simulink model "P_car"  (R2013b)
settings: Solver=ode45  StartTime=0.0  StopTime=10.0  RelTol=1e-3
values from neighbouring files (symbols this model uses):
  g = 9.81    [parameters.m]
  l_p = sqrt(0.115^2 + h_CG^2)    [parameters.m]
  l_w = 0.30    (= 0.3)    [parameters.m]    (also in testing.m = 0.4)
  m_car = 0.7    [dynamics_constants.m]    (also in parameters.m = 1.2)
  pf_mapping_1st_FR = polyfit(alphaF,beta_F,1)    [parameters.m]
  pf_mapping_1st_RR = mean(beta_R)    [parameters.m]
  v_R = 1 + 0.2*randn    [analyze_parameter_impcact.m]    (also in parameters.m = 1)
  w_w = 20    [parameters.m]
  w_z = 0.5    [parameters.m]
settings Model: Creator=daniel  LastModifiedBy=daniel

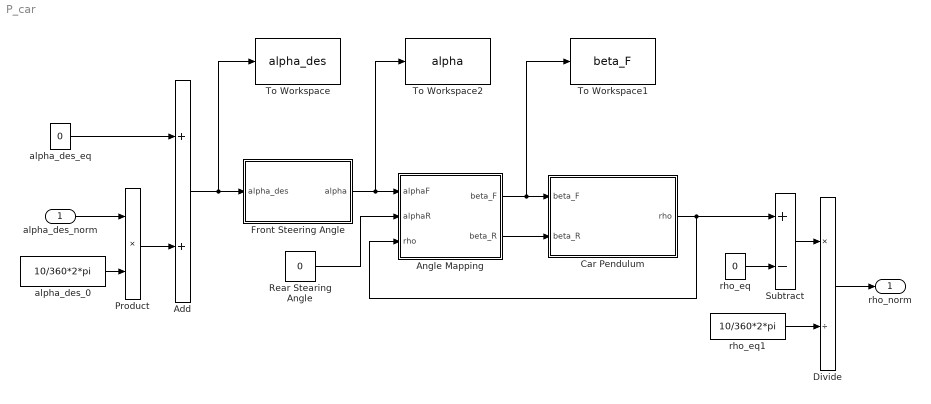
== system P_car ==
  alpha_des_norm : Inport
  Add : Sum
  Angle Mapping : Subsystem
  Car Pendulum : Subsystem
  Divide : Product  Inputs=*/
  Front Steering Angle : Subsystem
  Product : Product
  Rear Stearing Angle : Constant  Value=0
  Subtract : Sum  Inputs=+-
  To Workspace : ToWorkspace  VariableName=alpha_des  SampleTime=-1  SaveFormat=Timeseries
  To Workspace1 : ToWorkspace  VariableName=beta_F  SampleTime=-1  SaveFormat=Timeseries
  To Workspace2 : ToWorkspace  VariableName=alpha  SampleTime=-1  SaveFormat=Timeseries
  alpha_des_0 : Constant  Value=10/360*2*pi
  alpha_des_eq : Constant  Value=0
  rho_eq : Constant  Value=0
  rho_eq1 : Constant  Value=10/360*2*pi
  rho_norm : Outport
  wires:
  Car Pendulum/1(rho) -> Subtract/1, Angle Mapping/3(rho)
  Angle Mapping/2(beta_R) -> Car Pendulum/2(beta_R)
  Rear Stearing Angle/1 -> Angle Mapping/2(alphaR)
  Angle Mapping/1(beta_F) -> To Workspace1/1, Car Pendulum/1(beta_F)
  alpha_des_0/1 -> Product/2
  alpha_des_norm/1 -> Product/1
  Product/1 -> Add/2
  Add/1 -> To Workspace/1, Front Steering Angle/1(alpha_des)
  alpha_des_eq/1 -> Add/1
  rho_eq/1 -> Subtract/2
  Subtract/1 -> Divide/1
  rho_eq1/1 -> Divide/2
  Divide/1 -> rho_norm/1
  Front Steering Angle/1(alpha) -> To Workspace2/1, Angle Mapping/1(alphaF)

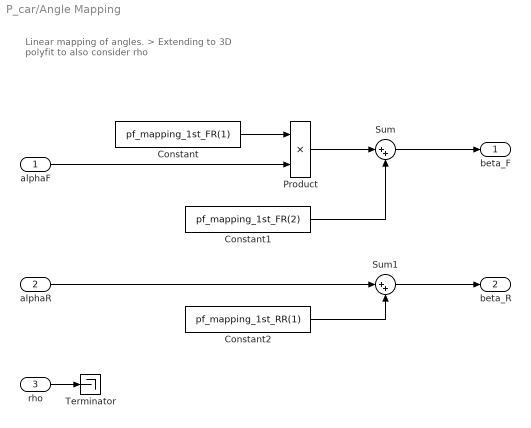
== system P_car/Angle Mapping ==
  note: Linear mapping of angles.
      |
      | > Extending to 3D polyfit to also consider rho
  alphaF : Inport
  alphaR : Inport  Port=2
  rho : Inport  Port=3
  Constant : Constant  Value=pf_mapping_1st_FR(1)
  Constant1 : Constant  Value=pf_mapping_1st_FR(2)
  Constant2 : Constant  Value=pf_mapping_1st_RR(1)
  Product : Product
  Sum : Sum  Inputs=|++
  Sum1 : Sum  Inputs=|++
  Terminator : Terminator
  beta_F : Outport
  beta_R : Outport  Port=2
  wires:
  Constant1/1 -> Sum/2
  Product/1 -> Sum/1
  Constant/1 -> Product/1
  alphaF/1 -> Product/2
  Sum/1 -> beta_F/1
  Sum1/1 -> beta_R/1
  alphaR/1 -> Sum1/1
  Constant2/1 -> Sum1/2
  rho/1 -> Terminator/1

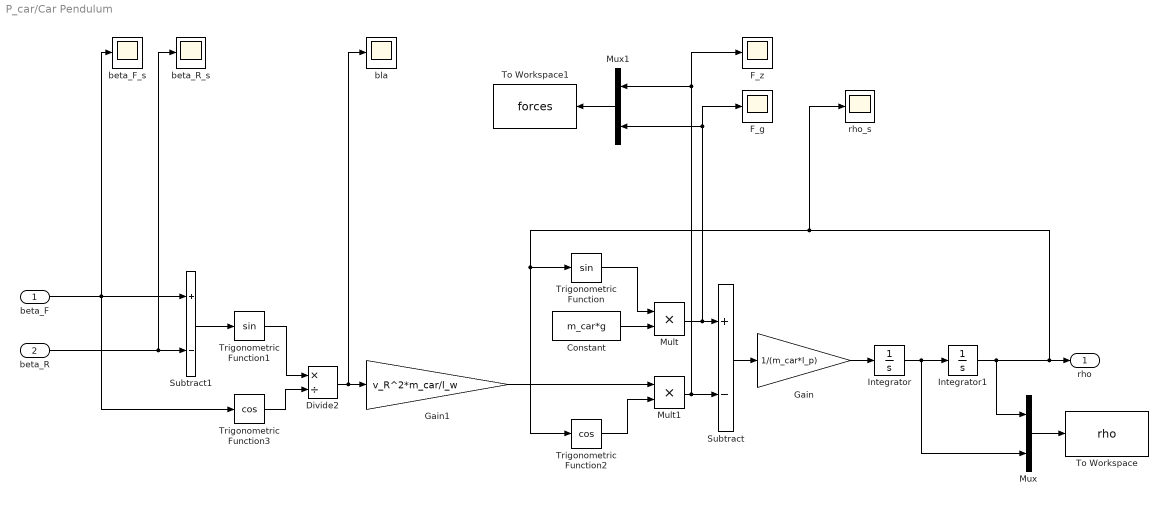
== system P_car/Car Pendulum ==
  beta_F : Inport
  beta_R : Inport  Port=2
  Constant : Constant  Value=m_car*g
  Divide2 : Product  Inputs=*/
  F_g : Scope
      settings: SaveName=ScopeData2
  F_z : Scope
  Gain : Gain  Gain=1/(m_car*l_p)
  Gain1 : Gain  Gain=v_R^2*m_car/l_w
  Integrator : Integrator  ContinuousStateAttributes='rho_dot'
  Integrator1 : Integrator  InitialCondition=2/360*2*pi*0  ContinuousStateAttributes='rho'
  Mult : Product  Inputs=**
  Mult1 : Product  Inputs=**
  Mux : Mux  Inputs=2
  Mux1 : Mux  Inputs=2
  Subtract : Sum  Inputs=+-
  Subtract1 : Sum  Inputs=+-
  To Workspace : ToWorkspace  VariableName=rho  SampleTime=-1  SaveFormat=Timeseries
  To Workspace1 : ToWorkspace  VariableName=forces  SampleTime=-1  SaveFormat=Timeseries
  Trigonometric Function : Trigonometry
  Trigonometric Function1 : Trigonometry
  Trigonometric Function2 : Trigonometry  Operator=cos
  Trigonometric Function3 : Trigonometry  Operator=cos
  beta_F_s : Scope
      settings: SaveName=ScopeData7
  "beta_R_s " : Scope
      settings: SaveName=ScopeData9
  bla : Scope
      settings: SaveName=ScopeData10
  rho_s : Scope
      settings: SaveName=ScopeData3
  rho : Outport
  wires:
  Integrator/1 -> Mux/2, Integrator1/1
  Mult1/1 -> F_z/1, Mux1/1, Subtract/2
  Mult/1 -> F_g/1, Mux1/2, Subtract/1
  beta_F/1 -> Trigonometric Function3/1, beta_F_s/1, Subtract1/1
  beta_R/1 -> "beta_R_s "/1, Subtract1/2
  Trigonometric Function1/1 -> Divide2/1
  Divide2/1 -> bla/1, Gain1/1
  Gain/1 -> Integrator/1
  Subtract/1 -> Gain/1
  Subtract1/1 -> Trigonometric Function1/1
  Mux/1 -> To Workspace/1
  Gain1/1 -> Mult1/1
  Constant/1 -> Mult/2
  Mux1/1 -> To Workspace1/1
  Trigonometric Function3/1 -> Divide2/2
  Integrator1/1 -> rho_s/1, Trigonometric Function/1, Trigonometric Function2/1, rho/1, Mux/1
  Trigonometric Function/1 -> Mult/1
  Trigonometric Function2/1 -> Mult1/2

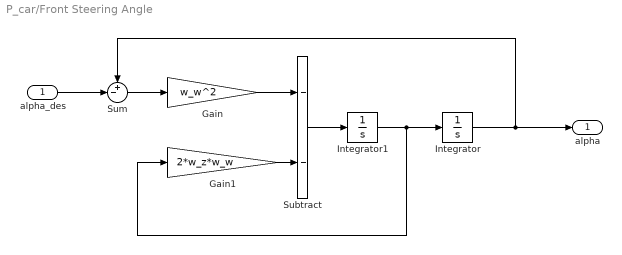
== system P_car/Front Steering Angle ==
  alpha_des : Inport
  Gain : Gain  Gain=w_w^2
  Gain1 : Gain  Gain=2*w_z*w_w
  Integrator : Integrator
  Integrator1 : Integrator
  Subtract : Sum  Inputs=--
  Sum : Sum  Inputs=+-|
  alpha : Outport
  wires:
  Integrator/1 -> alpha/1, Sum/1
  Subtract/1 -> Integrator1/1
  Sum/1 -> Gain/1
  Integrator1/1 -> Gain1/1, Integrator/1
  Gain/1 -> Subtract/1
  Gain1/1 -> Subtract/2
  alpha_des/1 -> Sum/2
